simulink model "Porblem_1"  (R2020a)
settings: Solver=VariableStepAuto  StartTime=0.0  StopTime=inf  RelTol=1e-3
settings Model: Creator=Shubham Singh Rathor  LastModifiedBy=Shubham Singh Rathor

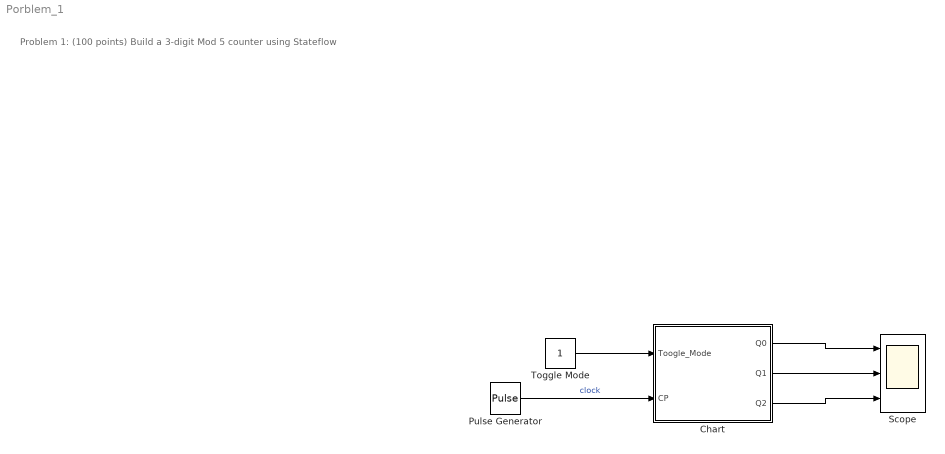
== system Porblem_1 ==
  note: Problem 1: (100 points) Build a 3-digit Mod 5 counter using Stateflow
  Chart : Stateflow chart  TreatAsAtomicUnit=on
  Pulse Generator : DiscretePulseGenerator  PulseType=Time based  Period=10  PulseWidth=5
  Scope : Scope  NumInputPorts=3
  Toggle Mode : Constant
  wires:
  Toggle Mode/1 -> Chart/1(Toogle_Mode)
  Chart/2(Q1) -> Scope/2
  Chart/1(Q0) -> Scope/1
  Chart/3(Q2) -> Scope/3
  Pulse Generator/1 -> Chart/2(CP)  "clock"

== stateflow chart Porblem_1/Chart ==
  state Init
    entry:
    Q0 = 0;
    Q1 = 0;
    Q2 = 0;
    state FF2
      entry:
      J2 = Toogle_Mode;
      K2 = Toogle_Mode;
      exit:
      flag = 1;
      during:
      (default) -> (junction 87) : % Toggling Q2
      (junction 87) -> (junction 88) [order 1] : [J2 == 1 && K2 == 1 && Q2 == 0 && Q1 == 1]
      (junction 87) -> (junction 89) [order 2]
      (junction 88) -> (junction 93) : {Q2 = 1;}
      (junction 89) -> (junction 90) [order 1] : [J2 == 1 && K2 == 1 && Q2 == 1 && Q1 == 1]
      (junction 89) -> (junction 91) [order 2]
      (junction 90) -> (junction 92) : {Q2 = 0;}
      (junction 92) -> (junction 91)
      (junction 93) -> (junction 92)
      (junction 91) -> (junction 94)
    state FF1
      entry:
      J1 = Toogle_Mode;
      K1 = Toogle_Mode;
      during:
      (default) -> (junction 69) : % Toggling Q1
      (junction 69) -> (junction 70) [order 1] : [J1 == 1 && K1 == 1 && Q1 == 0 && Q0 == 1]
      (junction 69) -> (junction 71) [order 2]
      (junction 70) -> (junction 75) : {Q1 = 1;}
      (junction 71) -> (junction 72) [order 1] : [J1 == 1 && K1 == 1 && Q1 == 1 && Q0]
      (junction 71) -> (junction 73) [order 2]
      (junction 72) -> (junction 74) : {Q1 = 0;}
      (junction 74) -> (junction 73)
      (junction 75) -> (junction 74)
      (junction 73) -> (junction 76)
    state FF0
      entry:
      J0 = Toogle_Mode;
      K0 = Toogle_Mode;
      clk = CP;
      flag = 0;
      during:
      (default) -> (junction 51) : % Toggling Q0
      (junction 51) -> (junction 52) [order 1] : [J0 == 1 &&  K0 == 1 && Q0 == 0 && clk == 1 ]
      (junction 51) -> (junction 53) [order 2]
      (junction 52) -> (junction 57) : {Q0 = 1;}
      (junction 53) -> (junction 54) [order 1] : [J0 == 1 &&  K0 == 1 && Q0 == 1 && clk == 1]
      (junction 53) -> (junction 55) [order 2]
      (junction 54) -> (junction 56) : {Q0 = 0;}
      (junction 56) -> (junction 55)
      (junction 57) -> (junction 56)
      (junction 55) -> (junction 58)
    (default) -> FF0
    FF1 -> FF2 : [Q1 ~= 0]
    FF0 -> FF1 : [Q0 ~= 0]
    FF2 -> FF0 : [flag == 1]
  (default) -> Init
  data: Toogle_Mode input; J0 local; J1 local; J2 local; K0 local; K1 local; K2 local; Q0 output; Q1 output; Q2 output; CP input; clk local; flag local
